simulink model "Systolic_4x4"  (R2021a)
settings: Solver=VariableStepAuto  StartTime=0.0  StopTime=32  RelTol=1e-3
libraries: hdlBasic x195, xbsIndex_r4 x1
(part 2 of 2)

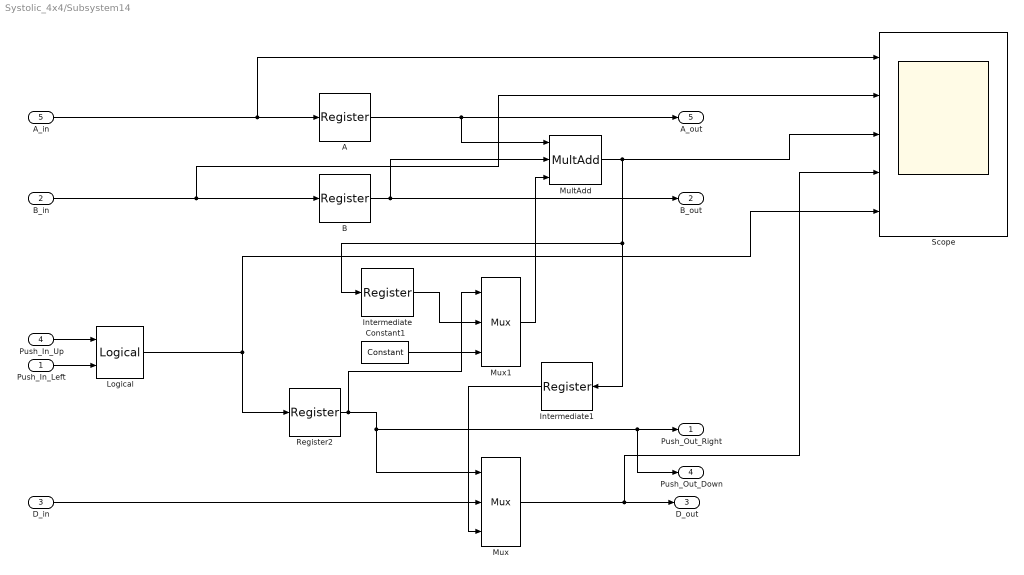
== system Systolic_4x4/Subsystem14 ==
  Push_In_Left : Inport
  B_in : Inport  Port=2
  D_in : Inport  Port=3
  Push_In_Up : Inport  Port=4
  A_in : Inport  Port=5
  A : hdlBasic/Register  init=0  rst=off  en=off  XmcBlockStatus=1  maskContainerNames=tabcontainer1  block_type=register  block_config=sysgen:Register_config
  B : hdlBasic/Register  init=0  rst=off  en=off  XmcBlockStatus=1  maskContainerNames=tabcontainer1  block_type=register  block_config=sysgen:Register_config
  Constant1 : hdlBasic/Constant  const=0  gui_display_data_type=Fixed-point  arith_type=Signed (2's comp)  n_bits=16  bin_pt=0  preci_type=Single  exp_width=8  frac_width=24  explicit_period=off  period=1  XmcBlockStatus=1  maskContainerNames=tabcontainer1  block_type=constant  block_config=sysgen:Constant_config
  Intermediate : hdlBasic/Register  init=0  rst=off  en=off  XmcBlockStatus=1  maskContainerNames=tabcontainer1  block_type=register  block_config=sysgen:Register_config
  Intermediate1 : hdlBasic/Register  init=0  rst=off  en=off  XmcBlockStatus=1  maskContainerNames=tabcontainer1  block_type=register  block_config=sysgen:Register_config
  Logical : hdlBasic/Logical  logical_function=OR  inputs=2  en=off  latency=0  precision=Full  arith_type=Unsigned  n_bits=16  bin_pt=0  align_bp=on  overflow=[]  quantization=[]  XmcBlockStatus=1  maskContainerNames=tabcontainer1  block_type=logical  block_config=sysgen:Logical_config
  MultAdd : hdlBasic/MultAdd  mode=Addition  en=off  latency=0  precision=Full  arith_type=Unsigned  n_bits=16  bin_pt=14  XmcBlockStatus=1  maskContainerNames=tabcontainer1  block_type=multadd  block_config=sysgen:MultAdd_config
  Mux : hdlBasic/Mux  inputs=2  en=off  latency=0  precision=User Defined  arith_type=Unsigned  n_bits=16  bin_pt=0  quantization=Truncate  overflow=Wrap  XmcBlockStatus=1  maskContainerNames=tabcontainer1  block_type=mux  block_config=sysgen:Mux_config
  Mux1 : hdlBasic/Mux  inputs=2  en=off  latency=0  precision=User Defined  arith_type=Unsigned  n_bits=16  bin_pt=0  quantization=Truncate  overflow=Wrap  XmcBlockStatus=1  maskContainerNames=tabcontainer1  block_type=mux  block_config=sysgen:Mux_config
  Register2 : hdlBasic/Register  init=0  rst=off  en=off  XmcBlockStatus=1  maskContainerNames=tabcontainer1  block_type=register  block_config=sysgen:Register_config
  Scope : Scope  NumInputPorts=5
  Push_Out_Right : Outport
  B_out : Outport  Port=2
  D_out : Outport  Port=3
  Push_Out_Down : Outport  Port=4
  A_out : Outport  Port=5
  wires:
  A/1 -> MultAdd/1, A_out/1
  B/1 -> MultAdd/2, B_out/1
  B_in/1 -> Scope/2, B/1
  A_in/1 -> Scope/1, A/1
  Mux/1 -> Scope/4, D_out/1
  D_in/1 -> Mux/2
  Push_In_Left/1 -> Logical/2
  Push_In_Up/1 -> Logical/1
  Register2/1 -> Mux1/1, Mux/1, Push_Out_Down/1, Push_Out_Right/1
  Logical/1 -> Scope/5, Register2/1
  Intermediate/1 -> Mux1/2
  Mux1/1 -> MultAdd/3
  Constant1/1 -> Mux1/3
  MultAdd/1 -> Scope/3, Intermediate1/1, Intermediate/1
  Intermediate1/1 -> Mux/3

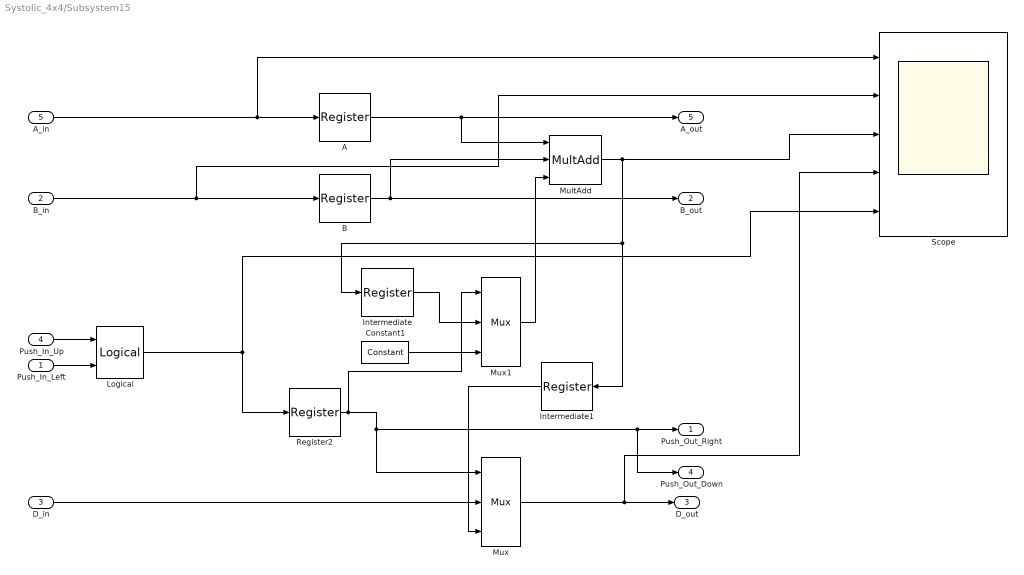
== system Systolic_4x4/Subsystem15 ==
  Push_In_Left : Inport
  B_in : Inport  Port=2
  D_in : Inport  Port=3
  Push_In_Up : Inport  Port=4
  A_in : Inport  Port=5
  A : hdlBasic/Register  init=0  rst=off  en=off  XmcBlockStatus=1  maskContainerNames=tabcontainer1  block_type=register  block_config=sysgen:Register_config
  B : hdlBasic/Register  init=0  rst=off  en=off  XmcBlockStatus=1  maskContainerNames=tabcontainer1  block_type=register  block_config=sysgen:Register_config
  Constant1 : hdlBasic/Constant  const=0  gui_display_data_type=Fixed-point  arith_type=Signed (2's comp)  n_bits=16  bin_pt=0  preci_type=Single  exp_width=8  frac_width=24  explicit_period=off  period=1  XmcBlockStatus=1  maskContainerNames=tabcontainer1  block_type=constant  block_config=sysgen:Constant_config
  Intermediate : hdlBasic/Register  init=0  rst=off  en=off  XmcBlockStatus=1  maskContainerNames=tabcontainer1  block_type=register  block_config=sysgen:Register_config
  Intermediate1 : hdlBasic/Register  init=0  rst=off  en=off  XmcBlockStatus=1  maskContainerNames=tabcontainer1  block_type=register  block_config=sysgen:Register_config
  Logical : hdlBasic/Logical  logical_function=OR  inputs=2  en=off  latency=0  precision=Full  arith_type=Unsigned  n_bits=16  bin_pt=0  align_bp=on  overflow=[]  quantization=[]  XmcBlockStatus=1  maskContainerNames=tabcontainer1  block_type=logical  block_config=sysgen:Logical_config
  MultAdd : hdlBasic/MultAdd  mode=Addition  en=off  latency=0  precision=Full  arith_type=Unsigned  n_bits=16  bin_pt=14  XmcBlockStatus=1  maskContainerNames=tabcontainer1  block_type=multadd  block_config=sysgen:MultAdd_config
  Mux : hdlBasic/Mux  inputs=2  en=off  latency=0  precision=User Defined  arith_type=Unsigned  n_bits=16  bin_pt=0  quantization=Truncate  overflow=Wrap  XmcBlockStatus=1  maskContainerNames=tabcontainer1  block_type=mux  block_config=sysgen:Mux_config
  Mux1 : hdlBasic/Mux  inputs=2  en=off  latency=0  precision=User Defined  arith_type=Unsigned  n_bits=16  bin_pt=0  quantization=Truncate  overflow=Wrap  XmcBlockStatus=1  maskContainerNames=tabcontainer1  block_type=mux  block_config=sysgen:Mux_config
  Register2 : hdlBasic/Register  init=0  rst=off  en=off  XmcBlockStatus=1  maskContainerNames=tabcontainer1  block_type=register  block_config=sysgen:Register_config
  Scope : Scope  NumInputPorts=5
  Push_Out_Right : Outport
  B_out : Outport  Port=2
  D_out : Outport  Port=3
  Push_Out_Down : Outport  Port=4
  A_out : Outport  Port=5
  wires:
  A/1 -> MultAdd/1, A_out/1
  B/1 -> MultAdd/2, B_out/1
  B_in/1 -> Scope/2, B/1
  A_in/1 -> Scope/1, A/1
  Mux/1 -> Scope/4, D_out/1
  D_in/1 -> Mux/2
  Push_In_Left/1 -> Logical/2
  Push_In_Up/1 -> Logical/1
  Register2/1 -> Mux1/1, Mux/1, Push_Out_Down/1, Push_Out_Right/1
  Logical/1 -> Scope/5, Register2/1
  Intermediate/1 -> Mux1/2
  Mux1/1 -> MultAdd/3
  Constant1/1 -> Mux1/3
  MultAdd/1 -> Scope/3, Intermediate1/1, Intermediate/1
  Intermediate1/1 -> Mux/3

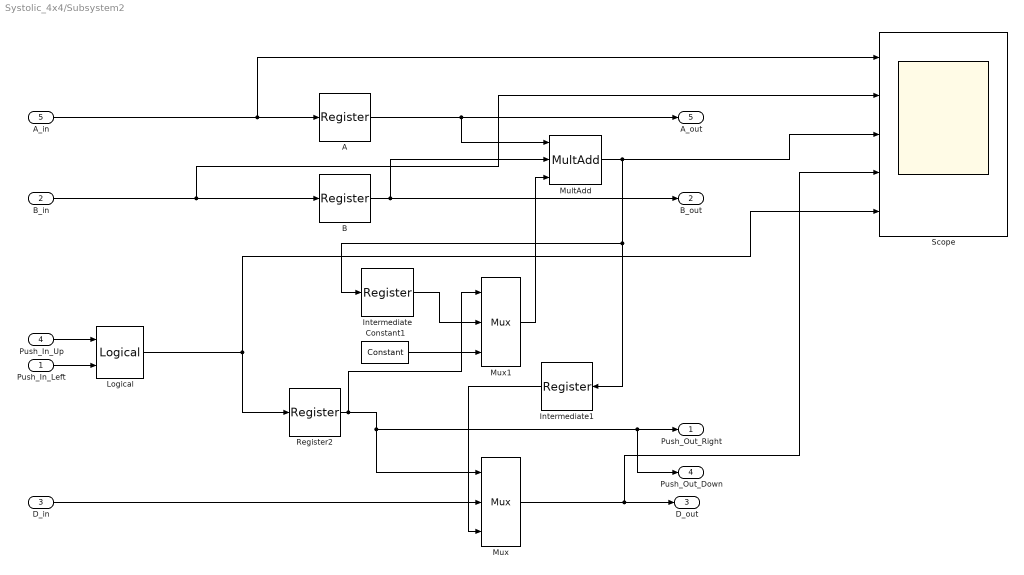
== system Systolic_4x4/Subsystem2 ==
  Push_In_Left : Inport
  B_in : Inport  Port=2
  D_in : Inport  Port=3
  Push_In_Up : Inport  Port=4
  A_in : Inport  Port=5
  A : hdlBasic/Register  init=0  rst=off  en=off  XmcBlockStatus=1  maskContainerNames=tabcontainer1  block_type=register  block_config=sysgen:Register_config
  B : hdlBasic/Register  init=0  rst=off  en=off  XmcBlockStatus=1  maskContainerNames=tabcontainer1  block_type=register  block_config=sysgen:Register_config
  Constant1 : hdlBasic/Constant  const=0  gui_display_data_type=Fixed-point  arith_type=Signed (2's comp)  n_bits=16  bin_pt=0  preci_type=Single  exp_width=8  frac_width=24  explicit_period=off  period=1  XmcBlockStatus=1  maskContainerNames=tabcontainer1  block_type=constant  block_config=sysgen:Constant_config
  Intermediate : hdlBasic/Register  init=0  rst=off  en=off  XmcBlockStatus=1  maskContainerNames=tabcontainer1  block_type=register  block_config=sysgen:Register_config
  Intermediate1 : hdlBasic/Register  init=0  rst=off  en=off  XmcBlockStatus=1  maskContainerNames=tabcontainer1  block_type=register  block_config=sysgen:Register_config
  Logical : hdlBasic/Logical  logical_function=OR  inputs=2  en=off  latency=0  precision=Full  arith_type=Unsigned  n_bits=16  bin_pt=0  align_bp=on  overflow=[]  quantization=[]  XmcBlockStatus=1  maskContainerNames=tabcontainer1  block_type=logical  block_config=sysgen:Logical_config
  MultAdd : hdlBasic/MultAdd  mode=Addition  en=off  latency=0  precision=Full  arith_type=Unsigned  n_bits=16  bin_pt=14  XmcBlockStatus=1  maskContainerNames=tabcontainer1  block_type=multadd  block_config=sysgen:MultAdd_config
  Mux : hdlBasic/Mux  inputs=2  en=off  latency=0  precision=User Defined  arith_type=Unsigned  n_bits=16  bin_pt=0  quantization=Truncate  overflow=Wrap  XmcBlockStatus=1  maskContainerNames=tabcontainer1  block_type=mux  block_config=sysgen:Mux_config
  Mux1 : hdlBasic/Mux  inputs=2  en=off  latency=0  precision=User Defined  arith_type=Unsigned  n_bits=16  bin_pt=0  quantization=Truncate  overflow=Wrap  XmcBlockStatus=1  maskContainerNames=tabcontainer1  block_type=mux  block_config=sysgen:Mux_config
  Register2 : hdlBasic/Register  init=0  rst=off  en=off  XmcBlockStatus=1  maskContainerNames=tabcontainer1  block_type=register  block_config=sysgen:Register_config
  Scope : Scope  NumInputPorts=5
  Push_Out_Right : Outport
  B_out : Outport  Port=2
  D_out : Outport  Port=3
  Push_Out_Down : Outport  Port=4
  A_out : Outport  Port=5
  wires:
  A/1 -> MultAdd/1, A_out/1
  B/1 -> MultAdd/2, B_out/1
  B_in/1 -> Scope/2, B/1
  A_in/1 -> Scope/1, A/1
  Mux/1 -> Scope/4, D_out/1
  D_in/1 -> Mux/2
  Push_In_Left/1 -> Logical/2
  Push_In_Up/1 -> Logical/1
  Register2/1 -> Mux1/1, Mux/1, Push_Out_Down/1, Push_Out_Right/1
  Logical/1 -> Scope/5, Register2/1
  Intermediate/1 -> Mux1/2
  Mux1/1 -> MultAdd/3
  Constant1/1 -> Mux1/3
  MultAdd/1 -> Scope/3, Intermediate1/1, Intermediate/1
  Intermediate1/1 -> Mux/3

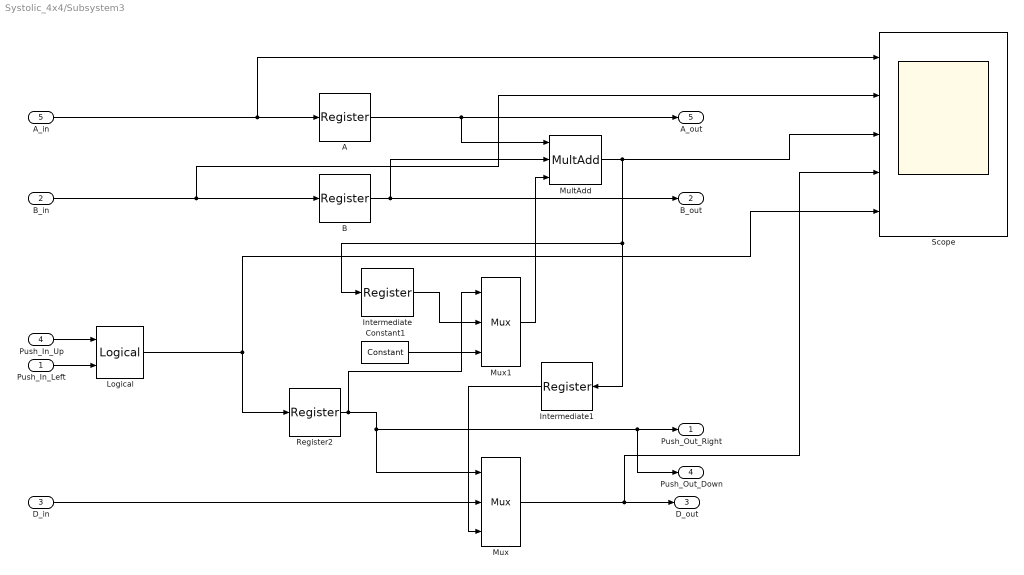
== system Systolic_4x4/Subsystem3 ==
  Push_In_Left : Inport
  B_in : Inport  Port=2
  D_in : Inport  Port=3
  Push_In_Up : Inport  Port=4
  A_in : Inport  Port=5
  A : hdlBasic/Register  init=0  rst=off  en=off  XmcBlockStatus=1  maskContainerNames=tabcontainer1  block_type=register  block_config=sysgen:Register_config
  B : hdlBasic/Register  init=0  rst=off  en=off  XmcBlockStatus=1  maskContainerNames=tabcontainer1  block_type=register  block_config=sysgen:Register_config
  Constant1 : hdlBasic/Constant  const=0  gui_display_data_type=Fixed-point  arith_type=Signed (2's comp)  n_bits=16  bin_pt=0  preci_type=Single  exp_width=8  frac_width=24  explicit_period=off  period=1  XmcBlockStatus=1  maskContainerNames=tabcontainer1  block_type=constant  block_config=sysgen:Constant_config
  Intermediate : hdlBasic/Register  init=0  rst=off  en=off  XmcBlockStatus=1  maskContainerNames=tabcontainer1  block_type=register  block_config=sysgen:Register_config
  Intermediate1 : hdlBasic/Register  init=0  rst=off  en=off  XmcBlockStatus=1  maskContainerNames=tabcontainer1  block_type=register  block_config=sysgen:Register_config
  Logical : hdlBasic/Logical  logical_function=OR  inputs=2  en=off  latency=0  precision=Full  arith_type=Unsigned  n_bits=16  bin_pt=0  align_bp=on  overflow=[]  quantization=[]  XmcBlockStatus=1  maskContainerNames=tabcontainer1  block_type=logical  block_config=sysgen:Logical_config
  MultAdd : hdlBasic/MultAdd  mode=Addition  en=off  latency=0  precision=Full  arith_type=Unsigned  n_bits=16  bin_pt=14  XmcBlockStatus=1  maskContainerNames=tabcontainer1  block_type=multadd  block_config=sysgen:MultAdd_config
  Mux : hdlBasic/Mux  inputs=2  en=off  latency=0  precision=User Defined  arith_type=Unsigned  n_bits=16  bin_pt=0  quantization=Truncate  overflow=Wrap  XmcBlockStatus=1  maskContainerNames=tabcontainer1  block_type=mux  block_config=sysgen:Mux_config
  Mux1 : hdlBasic/Mux  inputs=2  en=off  latency=0  precision=User Defined  arith_type=Unsigned  n_bits=16  bin_pt=0  quantization=Truncate  overflow=Wrap  XmcBlockStatus=1  maskContainerNames=tabcontainer1  block_type=mux  block_config=sysgen:Mux_config
  Register2 : hdlBasic/Register  init=0  rst=off  en=off  XmcBlockStatus=1  maskContainerNames=tabcontainer1  block_type=register  block_config=sysgen:Register_config
  Scope : Scope  NumInputPorts=5
  Push_Out_Right : Outport
  B_out : Outport  Port=2
  D_out : Outport  Port=3
  Push_Out_Down : Outport  Port=4
  A_out : Outport  Port=5
  wires:
  A/1 -> MultAdd/1, A_out/1
  B/1 -> MultAdd/2, B_out/1
  B_in/1 -> Scope/2, B/1
  A_in/1 -> Scope/1, A/1
  Mux/1 -> Scope/4, D_out/1
  D_in/1 -> Mux/2
  Push_In_Left/1 -> Logical/2
  Push_In_Up/1 -> Logical/1
  Register2/1 -> Mux1/1, Mux/1, Push_Out_Down/1, Push_Out_Right/1
  Logical/1 -> Scope/5, Register2/1
  Intermediate/1 -> Mux1/2
  Mux1/1 -> MultAdd/3
  Constant1/1 -> Mux1/3
  MultAdd/1 -> Scope/3, Intermediate1/1, Intermediate/1
  Intermediate1/1 -> Mux/3

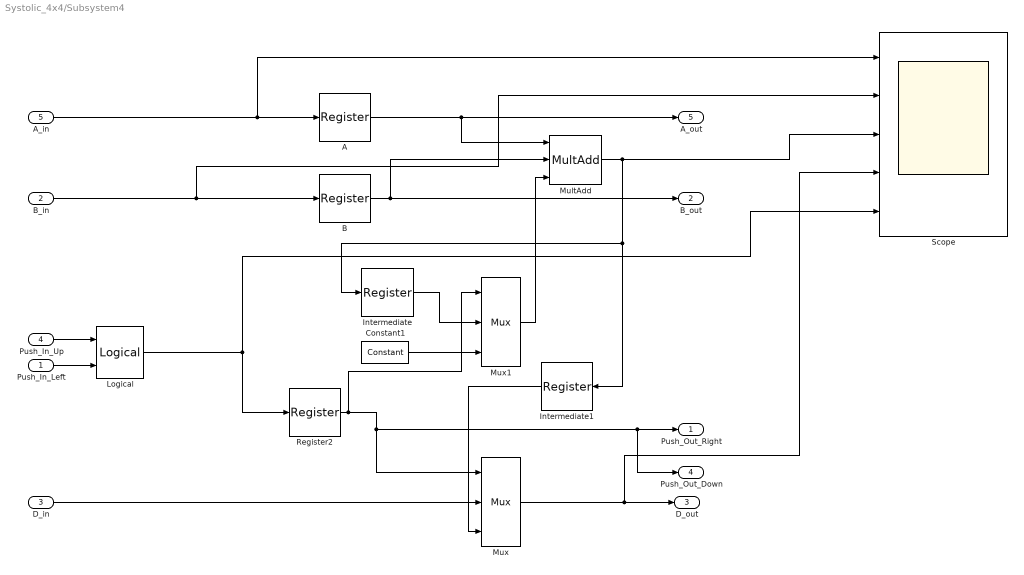
== system Systolic_4x4/Subsystem4 ==
  Push_In_Left : Inport
  B_in : Inport  Port=2
  D_in : Inport  Port=3
  Push_In_Up : Inport  Port=4
  A_in : Inport  Port=5
  A : hdlBasic/Register  init=0  rst=off  en=off  XmcBlockStatus=1  maskContainerNames=tabcontainer1  block_type=register  block_config=sysgen:Register_config
  B : hdlBasic/Register  init=0  rst=off  en=off  XmcBlockStatus=1  maskContainerNames=tabcontainer1  block_type=register  block_config=sysgen:Register_config
  Constant1 : hdlBasic/Constant  const=0  gui_display_data_type=Fixed-point  arith_type=Signed (2's comp)  n_bits=16  bin_pt=0  preci_type=Single  exp_width=8  frac_width=24  explicit_period=off  period=1  XmcBlockStatus=1  maskContainerNames=tabcontainer1  block_type=constant  block_config=sysgen:Constant_config
  Intermediate : hdlBasic/Register  init=0  rst=off  en=off  XmcBlockStatus=1  maskContainerNames=tabcontainer1  block_type=register  block_config=sysgen:Register_config
  Intermediate1 : hdlBasic/Register  init=0  rst=off  en=off  XmcBlockStatus=1  maskContainerNames=tabcontainer1  block_type=register  block_config=sysgen:Register_config
  Logical : hdlBasic/Logical  logical_function=OR  inputs=2  en=off  latency=0  precision=Full  arith_type=Unsigned  n_bits=16  bin_pt=0  align_bp=on  overflow=[]  quantization=[]  XmcBlockStatus=1  maskContainerNames=tabcontainer1  block_type=logical  block_config=sysgen:Logical_config
  MultAdd : hdlBasic/MultAdd  mode=Addition  en=off  latency=0  precision=Full  arith_type=Unsigned  n_bits=16  bin_pt=14  XmcBlockStatus=1  maskContainerNames=tabcontainer1  block_type=multadd  block_config=sysgen:MultAdd_config
  Mux : hdlBasic/Mux  inputs=2  en=off  latency=0  precision=User Defined  arith_type=Unsigned  n_bits=16  bin_pt=0  quantization=Truncate  overflow=Wrap  XmcBlockStatus=1  maskContainerNames=tabcontainer1  block_type=mux  block_config=sysgen:Mux_config
  Mux1 : hdlBasic/Mux  inputs=2  en=off  latency=0  precision=User Defined  arith_type=Unsigned  n_bits=16  bin_pt=0  quantization=Truncate  overflow=Wrap  XmcBlockStatus=1  maskContainerNames=tabcontainer1  block_type=mux  block_config=sysgen:Mux_config
  Register2 : hdlBasic/Register  init=0  rst=off  en=off  XmcBlockStatus=1  maskContainerNames=tabcontainer1  block_type=register  block_config=sysgen:Register_config
  Scope : Scope  NumInputPorts=5
  Push_Out_Right : Outport
  B_out : Outport  Port=2
  D_out : Outport  Port=3
  Push_Out_Down : Outport  Port=4
  A_out : Outport  Port=5
  wires:
  A/1 -> MultAdd/1, A_out/1
  B/1 -> MultAdd/2, B_out/1
  B_in/1 -> Scope/2, B/1
  A_in/1 -> Scope/1, A/1
  Mux/1 -> Scope/4, D_out/1
  D_in/1 -> Mux/2
  Push_In_Left/1 -> Logical/2
  Push_In_Up/1 -> Logical/1
  Register2/1 -> Mux1/1, Mux/1, Push_Out_Down/1, Push_Out_Right/1
  Logical/1 -> Scope/5, Register2/1
  Intermediate/1 -> Mux1/2
  Mux1/1 -> MultAdd/3
  Constant1/1 -> Mux1/3
  MultAdd/1 -> Scope/3, Intermediate1/1, Intermediate/1
  Intermediate1/1 -> Mux/3

== system Systolic_4x4/Subsystem5 ==
  Push_In_Left : Inport
  B_in : Inport  Port=2
  D_in : Inport  Port=3
  Push_In_Up : Inport  Port=4
  A_in : Inport  Port=5
  A : hdlBasic/Register  init=0  rst=off  en=off  XmcBlockStatus=1  maskContainerNames=tabcontainer1  block_type=register  block_config=sysgen:Register_config
  B : hdlBasic/Register  init=0  rst=off  en=off  XmcBlockStatus=1  maskContainerNames=tabcontainer1  block_type=register  block_config=sysgen:Register_config
  Constant1 : hdlBasic/Constant  const=0  gui_display_data_type=Fixed-point  arith_type=Signed (2's comp)  n_bits=16  bin_pt=0  preci_type=Single  exp_width=8  frac_width=24  explicit_period=off  period=1  XmcBlockStatus=1  maskContainerNames=tabcontainer1  block_type=constant  block_config=sysgen:Constant_config
  Intermediate : hdlBasic/Register  init=0  rst=off  en=off  XmcBlockStatus=1  maskContainerNames=tabcontainer1  block_type=register  block_config=sysgen:Register_config
  Intermediate1 : hdlBasic/Register  init=0  rst=off  en=off  XmcBlockStatus=1  maskContainerNames=tabcontainer1  block_type=register  block_config=sysgen:Register_config
  Logical : hdlBasic/Logical  logical_function=OR  inputs=2  en=off  latency=0  precision=Full  arith_type=Unsigned  n_bits=16  bin_pt=0  align_bp=on  overflow=[]  quantization=[]  XmcBlockStatus=1  maskContainerNames=tabcontainer1  block_type=logical  block_config=sysgen:Logical_config
  MultAdd : hdlBasic/MultAdd  mode=Addition  en=off  latency=0  precision=Full  arith_type=Unsigned  n_bits=16  bin_pt=14  XmcBlockStatus=1  maskContainerNames=tabcontainer1  block_type=multadd  block_config=sysgen:MultAdd_config
  Mux : hdlBasic/Mux  inputs=2  en=off  latency=0  precision=User Defined  arith_type=Unsigned  n_bits=16  bin_pt=0  quantization=Truncate  overflow=Wrap  XmcBlockStatus=1  maskContainerNames=tabcontainer1  block_type=mux  block_config=sysgen:Mux_config
  Mux1 : hdlBasic/Mux  inputs=2  en=off  latency=0  precision=User Defined  arith_type=Unsigned  n_bits=16  bin_pt=0  quantization=Truncate  overflow=Wrap  XmcBlockStatus=1  maskContainerNames=tabcontainer1  block_type=mux  block_config=sysgen:Mux_config
  Register2 : hdlBasic/Register  init=0  rst=off  en=off  XmcBlockStatus=1  maskContainerNames=tabcontainer1  block_type=register  block_config=sysgen:Register_config
  Scope : Scope  NumInputPorts=5
  Push_Out_Right : Outport
  B_out : Outport  Port=2
  D_out : Outport  Port=3
  Push_Out_Down : Outport  Port=4
  A_out : Outport  Port=5
  wires:
  A/1 -> MultAdd/1, A_out/1
  B/1 -> MultAdd/2, B_out/1
  B_in/1 -> Scope/2, B/1
  A_in/1 -> Scope/1, A/1
  Mux/1 -> Scope/4, D_out/1
  D_in/1 -> Mux/2
  Push_In_Left/1 -> Logical/2
  Push_In_Up/1 -> Logical/1
  Register2/1 -> Mux1/1, Mux/1, Push_Out_Down/1, Push_Out_Right/1
  Logical/1 -> Scope/5, Register2/1
  Intermediate/1 -> Mux1/2
  Mux1/1 -> MultAdd/3
  Constant1/1 -> Mux1/3
  MultAdd/1 -> Scope/3, Intermediate1/1, Intermediate/1
  Intermediate1/1 -> Mux/3

== system Systolic_4x4/Subsystem6 ==
  Push_In_Left : Inport
  B_in : Inport  Port=2
  D_in : Inport  Port=3
  Push_In_Up : Inport  Port=4
  A_in : Inport  Port=5
  A : hdlBasic/Register  init=0  rst=off  en=off  XmcBlockStatus=1  maskContainerNames=tabcontainer1  block_type=register  block_config=sysgen:Register_config
  B : hdlBasic/Register  init=0  rst=off  en=off  XmcBlockStatus=1  maskContainerNames=tabcontainer1  block_type=register  block_config=sysgen:Register_config
  Constant1 : hdlBasic/Constant  const=0  gui_display_data_type=Fixed-point  arith_type=Signed (2's comp)  n_bits=16  bin_pt=0  preci_type=Single  exp_width=8  frac_width=24  explicit_period=off  period=1  XmcBlockStatus=1  maskContainerNames=tabcontainer1  block_type=constant  block_config=sysgen:Constant_config
  Intermediate : hdlBasic/Register  init=0  rst=off  en=off  XmcBlockStatus=1  maskContainerNames=tabcontainer1  block_type=register  block_config=sysgen:Register_config
  Intermediate1 : hdlBasic/Register  init=0  rst=off  en=off  XmcBlockStatus=1  maskContainerNames=tabcontainer1  block_type=register  block_config=sysgen:Register_config
  Logical : hdlBasic/Logical  logical_function=OR  inputs=2  en=off  latency=0  precision=Full  arith_type=Unsigned  n_bits=16  bin_pt=0  align_bp=on  overflow=[]  quantization=[]  XmcBlockStatus=1  maskContainerNames=tabcontainer1  block_type=logical  block_config=sysgen:Logical_config
  MultAdd : hdlBasic/MultAdd  mode=Addition  en=off  latency=0  precision=Full  arith_type=Unsigned  n_bits=16  bin_pt=14  XmcBlockStatus=1  maskContainerNames=tabcontainer1  block_type=multadd  block_config=sysgen:MultAdd_config
  Mux : hdlBasic/Mux  inputs=2  en=off  latency=0  precision=User Defined  arith_type=Unsigned  n_bits=16  bin_pt=0  quantization=Truncate  overflow=Wrap  XmcBlockStatus=1  maskContainerNames=tabcontainer1  block_type=mux  block_config=sysgen:Mux_config
  Mux1 : hdlBasic/Mux  inputs=2  en=off  latency=0  precision=User Defined  arith_type=Unsigned  n_bits=16  bin_pt=0  quantization=Truncate  overflow=Wrap  XmcBlockStatus=1  maskContainerNames=tabcontainer1  block_type=mux  block_config=sysgen:Mux_config
  Register2 : hdlBasic/Register  init=0  rst=off  en=off  XmcBlockStatus=1  maskContainerNames=tabcontainer1  block_type=register  block_config=sysgen:Register_config
  Scope : Scope  NumInputPorts=5
  Push_Out_Right : Outport
  B_out : Outport  Port=2
  D_out : Outport  Port=3
  Push_Out_Down : Outport  Port=4
  A_out : Outport  Port=5
  wires:
  A/1 -> MultAdd/1, A_out/1
  B/1 -> MultAdd/2, B_out/1
  B_in/1 -> Scope/2, B/1
  A_in/1 -> Scope/1, A/1
  Mux/1 -> Scope/4, D_out/1
  D_in/1 -> Mux/2
  Push_In_Left/1 -> Logical/2
  Push_In_Up/1 -> Logical/1
  Register2/1 -> Mux1/1, Mux/1, Push_Out_Down/1, Push_Out_Right/1
  Logical/1 -> Scope/5, Register2/1
  Intermediate/1 -> Mux1/2
  Mux1/1 -> MultAdd/3
  Constant1/1 -> Mux1/3
  MultAdd/1 -> Scope/3, Intermediate1/1, Intermediate/1
  Intermediate1/1 -> Mux/3

== system Systolic_4x4/Subsystem7 ==
  Push_In_Left : Inport
  B_in : Inport  Port=2
  D_in : Inport  Port=3
  Push_In_Up : Inport  Port=4
  A_in : Inport  Port=5
  A : hdlBasic/Register  init=0  rst=off  en=off  XmcBlockStatus=1  maskContainerNames=tabcontainer1  block_type=register  block_config=sysgen:Register_config
  B : hdlBasic/Register  init=0  rst=off  en=off  XmcBlockStatus=1  maskContainerNames=tabcontainer1  block_type=register  block_config=sysgen:Register_config
  Constant1 : hdlBasic/Constant  const=0  gui_display_data_type=Fixed-point  arith_type=Signed (2's comp)  n_bits=16  bin_pt=0  preci_type=Single  exp_width=8  frac_width=24  explicit_period=off  period=1  XmcBlockStatus=1  maskContainerNames=tabcontainer1  block_type=constant  block_config=sysgen:Constant_config
  Intermediate : hdlBasic/Register  init=0  rst=off  en=off  XmcBlockStatus=1  maskContainerNames=tabcontainer1  block_type=register  block_config=sysgen:Register_config
  Intermediate1 : hdlBasic/Register  init=0  rst=off  en=off  XmcBlockStatus=1  maskContainerNames=tabcontainer1  block_type=register  block_config=sysgen:Register_config
  Logical : hdlBasic/Logical  logical_function=OR  inputs=2  en=off  latency=0  precision=Full  arith_type=Unsigned  n_bits=16  bin_pt=0  align_bp=on  overflow=[]  quantization=[]  XmcBlockStatus=1  maskContainerNames=tabcontainer1  block_type=logical  block_config=sysgen:Logical_config
  MultAdd : hdlBasic/MultAdd  mode=Addition  en=off  latency=0  precision=Full  arith_type=Unsigned  n_bits=16  bin_pt=14  XmcBlockStatus=1  maskContainerNames=tabcontainer1  block_type=multadd  block_config=sysgen:MultAdd_config
  Mux : hdlBasic/Mux  inputs=2  en=off  latency=0  precision=User Defined  arith_type=Unsigned  n_bits=16  bin_pt=0  quantization=Truncate  overflow=Wrap  XmcBlockStatus=1  maskContainerNames=tabcontainer1  block_type=mux  block_config=sysgen:Mux_config
  Mux1 : hdlBasic/Mux  inputs=2  en=off  latency=0  precision=User Defined  arith_type=Unsigned  n_bits=16  bin_pt=0  quantization=Truncate  overflow=Wrap  XmcBlockStatus=1  maskContainerNames=tabcontainer1  block_type=mux  block_config=sysgen:Mux_config
  Register2 : hdlBasic/Register  init=0  rst=off  en=off  XmcBlockStatus=1  maskContainerNames=tabcontainer1  block_type=register  block_config=sysgen:Register_config
  Scope : Scope  NumInputPorts=5
  Push_Out_Right : Outport
  B_out : Outport  Port=2
  D_out : Outport  Port=3
  Push_Out_Down : Outport  Port=4
  A_out : Outport  Port=5
  wires:
  A/1 -> MultAdd/1, A_out/1
  B/1 -> MultAdd/2, B_out/1
  B_in/1 -> Scope/2, B/1
  A_in/1 -> Scope/1, A/1
  Mux/1 -> Scope/4, D_out/1
  D_in/1 -> Mux/2
  Push_In_Left/1 -> Logical/2
  Push_In_Up/1 -> Logical/1
  Register2/1 -> Mux1/1, Mux/1, Push_Out_Down/1, Push_Out_Right/1
  Logical/1 -> Scope/5, Register2/1
  Intermediate/1 -> Mux1/2
  Mux1/1 -> MultAdd/3
  Constant1/1 -> Mux1/3
  MultAdd/1 -> Scope/3, Intermediate1/1, Intermediate/1
  Intermediate1/1 -> Mux/3

== system Systolic_4x4/Subsystem8 ==
  Push_In_Left : Inport
  B_in : Inport  Port=2
  D_in : Inport  Port=3
  Push_In_Up : Inport  Port=4
  A_in : Inport  Port=5
  A : hdlBasic/Register  init=0  rst=off  en=off  XmcBlockStatus=1  maskContainerNames=tabcontainer1  block_type=register  block_config=sysgen:Register_config
  B : hdlBasic/Register  init=0  rst=off  en=off  XmcBlockStatus=1  maskContainerNames=tabcontainer1  block_type=register  block_config=sysgen:Register_config
  Constant1 : hdlBasic/Constant  const=0  gui_display_data_type=Fixed-point  arith_type=Signed (2's comp)  n_bits=16  bin_pt=0  preci_type=Single  exp_width=8  frac_width=24  explicit_period=off  period=1  XmcBlockStatus=1  maskContainerNames=tabcontainer1  block_type=constant  block_config=sysgen:Constant_config
  Intermediate : hdlBasic/Register  init=0  rst=off  en=off  XmcBlockStatus=1  maskContainerNames=tabcontainer1  block_type=register  block_config=sysgen:Register_config
  Intermediate1 : hdlBasic/Register  init=0  rst=off  en=off  XmcBlockStatus=1  maskContainerNames=tabcontainer1  block_type=register  block_config=sysgen:Register_config
  Logical : hdlBasic/Logical  logical_function=OR  inputs=2  en=off  latency=0  precision=Full  arith_type=Unsigned  n_bits=16  bin_pt=0  align_bp=on  overflow=[]  quantization=[]  XmcBlockStatus=1  maskContainerNames=tabcontainer1  block_type=logical  block_config=sysgen:Logical_config
  MultAdd : hdlBasic/MultAdd  mode=Addition  en=off  latency=0  precision=Full  arith_type=Unsigned  n_bits=16  bin_pt=14  XmcBlockStatus=1  maskContainerNames=tabcontainer1  block_type=multadd  block_config=sysgen:MultAdd_config
  Mux : hdlBasic/Mux  inputs=2  en=off  latency=0  precision=User Defined  arith_type=Unsigned  n_bits=16  bin_pt=0  quantization=Truncate  overflow=Wrap  XmcBlockStatus=1  maskContainerNames=tabcontainer1  block_type=mux  block_config=sysgen:Mux_config
  Mux1 : hdlBasic/Mux  inputs=2  en=off  latency=0  precision=User Defined  arith_type=Unsigned  n_bits=16  bin_pt=0  quantization=Truncate  overflow=Wrap  XmcBlockStatus=1  maskContainerNames=tabcontainer1  block_type=mux  block_config=sysgen:Mux_config
  Register2 : hdlBasic/Register  init=0  rst=off  en=off  XmcBlockStatus=1  maskContainerNames=tabcontainer1  block_type=register  block_config=sysgen:Register_config
  Scope : Scope  NumInputPorts=5
  Push_Out_Right : Outport
  B_out : Outport  Port=2
  D_out : Outport  Port=3
  Push_Out_Down : Outport  Port=4
  A_out : Outport  Port=5
  wires:
  A/1 -> MultAdd/1, A_out/1
  B/1 -> MultAdd/2, B_out/1
  B_in/1 -> Scope/2, B/1
  A_in/1 -> Scope/1, A/1
  Mux/1 -> Scope/4, D_out/1
  D_in/1 -> Mux/2
  Push_In_Left/1 -> Logical/2
  Push_In_Up/1 -> Logical/1
  Register2/1 -> Mux1/1, Mux/1, Push_Out_Down/1, Push_Out_Right/1
  Logical/1 -> Scope/5, Register2/1
  Intermediate/1 -> Mux1/2
  Mux1/1 -> MultAdd/3
  Constant1/1 -> Mux1/3
  MultAdd/1 -> Scope/3, Intermediate1/1, Intermediate/1
  Intermediate1/1 -> Mux/3

== system Systolic_4x4/Subsystem9 ==
  Push_In_Left : Inport
  B_in : Inport  Port=2
  D_in : Inport  Port=3
  Push_In_Up : Inport  Port=4
  A_in : Inport  Port=5
  A : hdlBasic/Register  init=0  rst=off  en=off  XmcBlockStatus=1  maskContainerNames=tabcontainer1  block_type=register  block_config=sysgen:Register_config
  B : hdlBasic/Register  init=0  rst=off  en=off  XmcBlockStatus=1  maskContainerNames=tabcontainer1  block_type=register  block_config=sysgen:Register_config
  Constant1 : hdlBasic/Constant  const=0  gui_display_data_type=Fixed-point  arith_type=Signed (2's comp)  n_bits=16  bin_pt=0  preci_type=Single  exp_width=8  frac_width=24  explicit_period=off  period=1  XmcBlockStatus=1  maskContainerNames=tabcontainer1  block_type=constant  block_config=sysgen:Constant_config
  Intermediate : hdlBasic/Register  init=0  rst=off  en=off  XmcBlockStatus=1  maskContainerNames=tabcontainer1  block_type=register  block_config=sysgen:Register_config
  Intermediate1 : hdlBasic/Register  init=0  rst=off  en=off  XmcBlockStatus=1  maskContainerNames=tabcontainer1  block_type=register  block_config=sysgen:Register_config
  Logical : hdlBasic/Logical  logical_function=OR  inputs=2  en=off  latency=0  precision=Full  arith_type=Unsigned  n_bits=16  bin_pt=0  align_bp=on  overflow=[]  quantization=[]  XmcBlockStatus=1  maskContainerNames=tabcontainer1  block_type=logical  block_config=sysgen:Logical_config
  MultAdd : hdlBasic/MultAdd  mode=Addition  en=off  latency=0  precision=Full  arith_type=Unsigned  n_bits=16  bin_pt=14  XmcBlockStatus=1  maskContainerNames=tabcontainer1  block_type=multadd  block_config=sysgen:MultAdd_config
  Mux : hdlBasic/Mux  inputs=2  en=off  latency=0  precision=User Defined  arith_type=Unsigned  n_bits=16  bin_pt=0  quantization=Truncate  overflow=Wrap  XmcBlockStatus=1  maskContainerNames=tabcontainer1  block_type=mux  block_config=sysgen:Mux_config
  Mux1 : hdlBasic/Mux  inputs=2  en=off  latency=0  precision=User Defined  arith_type=Unsigned  n_bits=16  bin_pt=0  quantization=Truncate  overflow=Wrap  XmcBlockStatus=1  maskContainerNames=tabcontainer1  block_type=mux  block_config=sysgen:Mux_config
  Register2 : hdlBasic/Register  init=0  rst=off  en=off  XmcBlockStatus=1  maskContainerNames=tabcontainer1  block_type=register  block_config=sysgen:Register_config
  Scope : Scope  NumInputPorts=5
  Push_Out_Right : Outport
  B_out : Outport  Port=2
  D_out : Outport  Port=3
  Push_Out_Down : Outport  Port=4
  A_out : Outport  Port=5
  wires:
  A/1 -> MultAdd/1, A_out/1
  B/1 -> MultAdd/2, B_out/1
  B_in/1 -> Scope/2, B/1
  A_in/1 -> Scope/1, A/1
  Mux/1 -> Scope/4, D_out/1
  D_in/1 -> Mux/2
  Push_In_Left/1 -> Logical/2
  Push_In_Up/1 -> Logical/1
  Register2/1 -> Mux1/1, Mux/1, Push_Out_Down/1, Push_Out_Right/1
  Logical/1 -> Scope/5, Register2/1
  Intermediate/1 -> Mux1/2
  Mux1/1 -> MultAdd/3
  Constant1/1 -> Mux1/3
  MultAdd/1 -> Scope/3, Intermediate1/1, Intermediate/1
  Intermediate1/1 -> Mux/3
